simulink model "BaseEngineController_LS"  (Simulink 7.7)
settings: Solver=FixedStepDiscrete  StartTime=0.0  StopTime=10.0  RelTol=1e-3
PreLoadFcn:
  | try, eval([bdroot '_setup']); catch, eval('model_setup', ''); end
InitFcn:
  | try, eval([bdroot '_setup']); catch, eval('model_setup', ''); end
undefined symbols (not defined in the file): ECU555, High, motohawk_build_version, motohawk_trunc_name, motohawk_vardec_config_group, motohawk_vardec_path, True
libraries: MotoHawk_lib x1418, motohawk_control_primitives_lib x183, motohawk_engine_lib x32, simulink x21, motohawk_annotations_lib x9, AutoDoc_lib x8, simulink_extras x4, motohawk_ccp_examples_lib x1, motohawk_control_primitives_motoshare_lib x1
(part 17 of 27)

== system BaseEngineController_LS/Foreground/Control/VirtualSensors/RawProcessed/Capture ECT At Startup ==
  Signal_In : Inport
  Enable : EnablePort  StatesWhenEnabling=reset
  Add : Sum
  Add1 : Sum  Inputs=+-
  Collect Average : Subsystem  TreatAsAtomicUnit=on
  Constant : Constant  Value=int8(1)  SampleTime=-1
  Logical Operator : Logic  AllPortsSameDT=off  OutDataTypeStr=boolean
  Relational Operator : RelationalOperator  Operator=<=
  Relational Operator1 : RelationalOperator  Operator=>
  Sum : Sum  Inputs=++|  InputSameDT=on
  Switch : Switch  Threshold=1  ZeroCross=off  InputSameDT=on
  TwoSampleBuffer ToIgnore : Constant  Value=2  OutDataTypeStr=Inherit: Inherit via back propagation  SampleTime=-1
  Unit Delay : UnitDelay  SampleTime=-1
  motohawk_calibration : MotoHawk_lib/Calibration & Probing Blocks/motohawk_calibration  nam=[nam '_Count']  val=int8(count)  storage=Calibration  show_more=on  name_source=Use Parameter  data_type=Inherit from 'Default Value'  read_level=1  write_level=1  ovr_cals=on  view_as=Number  enum_struct={'Disabled', 'Enabled'}  vector_style=Wide Row  use_help_units=on  help='Number of samples to average at key-up to produce signal value'  units=''  use_header_enum=off  row_header_enum={}  col_header_enum={}  use_min_max=off  min_val=-inf  max_val=inf  use_precision=off  precision=''  gain=1  offset=0  exp=1  use_mototune_group=on  mototune_group=motohawk_vardec_path(gcb)
  motohawk_probe : MotoHawk_lib/Calibration & Probing Blocks/motohawk_probe  nam=nam  show_more=on  name_source=Use Parameter  read_level=1  view_as=Number  enum_struct={'Disabled', 'Enabled'}  vector_style=Wide Row  use_help_units=on  help=''  units=units  use_header_enum=off  row_header_enum={}  col_header_enum={}  use_precision=off  precision=''  gain=1  offset=0  exp=1  use_mototune_group=on  mototune_group=grp
  Signal_KeyUp : Outport
  wires:
  Sum/1 -> Switch/1, Relational Operator/1, Relational Operator1/1
  Relational Operator/1 -> Switch/2, Logical Operator/1
  Switch/1 -> Unit Delay/1, Add1/1
  Collect Average/1(Captured_Signal) -> motohawk_probe/1, Signal_KeyUp/1
  Signal_In/1 -> Collect Average/2(Signal)
  Unit Delay/1 -> Sum/1
  Constant/1 -> Sum/2
  motohawk_calibration/1 -> Add/1
  Add/1 -> Relational Operator/2, Switch/3
  TwoSampleBuffer ToIgnore/1 -> Add/2, Relational Operator1/2, Add1/2
  Logical Operator/1 -> Collect Average/Enable
  Relational Operator1/1 -> Logical Operator/2
  Add1/1 -> Collect Average/1(Count)

== system BaseEngineController_LS/Foreground/Control/VirtualSensors/RawProcessed/Capture IAT At Startup ==
  Signal_In : Inport
  Enable : EnablePort  StatesWhenEnabling=reset
  Add : Sum
  Add1 : Sum  Inputs=+-
  Collect Average : Subsystem  TreatAsAtomicUnit=on
  Constant : Constant  Value=int8(1)  SampleTime=-1
  Logical Operator : Logic  AllPortsSameDT=off  OutDataTypeStr=boolean
  Relational Operator : RelationalOperator  Operator=<=
  Relational Operator1 : RelationalOperator  Operator=>
  Sum : Sum  Inputs=++|  InputSameDT=on
  Switch : Switch  Threshold=1  ZeroCross=off  InputSameDT=on
  TwoSampleBuffer ToIgnore : Constant  Value=2  OutDataTypeStr=Inherit: Inherit via back propagation  SampleTime=-1
  Unit Delay : UnitDelay  SampleTime=-1
  motohawk_calibration : MotoHawk_lib/Calibration & Probing Blocks/motohawk_calibration  nam=[nam '_Count']  val=int8(count)  storage=Calibration  show_more=on  name_source=Use Parameter  data_type=Inherit from 'Default Value'  read_level=1  write_level=1  ovr_cals=on  view_as=Number  enum_struct={'Disabled', 'Enabled'}  vector_style=Wide Row  use_help_units=on  help='Number of samples to average at key-up to produce signal value'  units=''  use_header_enum=off  row_header_enum={}  col_header_enum={}  use_min_max=off  min_val=-inf  max_val=inf  use_precision=off  precision=''  gain=1  offset=0  exp=1  use_mototune_group=on  mototune_group=motohawk_vardec_path(gcb)
  motohawk_probe : MotoHawk_lib/Calibration & Probing Blocks/motohawk_probe  nam=nam  show_more=on  name_source=Use Parameter  read_level=1  view_as=Number  enum_struct={'Disabled', 'Enabled'}  vector_style=Wide Row  use_help_units=on  help=''  units=units  use_header_enum=off  row_header_enum={}  col_header_enum={}  use_precision=off  precision=''  gain=1  offset=0  exp=1  use_mototune_group=on  mototune_group=motohawk_vardec_path(gcb)
  Signal_KeyUp : Outport
  wires:
  Add1/1 -> Collect Average/1(Count)
  Relational Operator1/1 -> Logical Operator/2
  Logical Operator/1 -> Collect Average/Enable
  TwoSampleBuffer ToIgnore/1 -> Add1/2, Relational Operator1/2, Add/2
  Add/1 -> Switch/3, Relational Operator/2
  motohawk_calibration/1 -> Add/1
  Constant/1 -> Sum/2
  Unit Delay/1 -> Sum/1
  Signal_In/1 -> Collect Average/2(Signal)
  Collect Average/1(Captured_Signal) -> Signal_KeyUp/1, motohawk_probe/1
  Switch/1 -> Add1/1, Unit Delay/1
  Relational Operator/1 -> Logical Operator/1, Switch/2
  Sum/1 -> Relational Operator1/1, Relational Operator/1, Switch/1

== system BaseEngineController_LS/Foreground/Control/VirtualSensors/RawProcessed/CutThrottle APP Limiting ==
  APP_in [%] : Inport
  Bound APP if overheating : motohawk_control_primitives_lib/Saturation  SystemSampleTime=-1
  Constant1 : Constant  Value=0  SampleTime=-1
  Data Type Conversion : DataTypeConversion  OutDataTypeStr=double
  Product1 : Product  RndMeth=Zero
  Switch1 : Switch  Threshold=1
  motohawk_calibration1 : MotoHawk_lib/Calibration & Probing Blocks/motohawk_calibration  nam='Overheat_MaxAPP'  val=10  storage=Calibration  show_more=on  name_source=Use Parameter  data_type=uint8  read_level=1  write_level=1  ovr_cals=on  view_as=Number  enum_struct={'Disabled', 'Enabled'}  vector_style=Wide Row  use_help_units=on  help='Max APP command to allow during overheat condition'  units='%'  use_header_enum=off  row_header_enum={}  col_header_enum={}  use_min_max=on  min_val=-inf  max_val=inf  use_precision=off  precision=''  gain=1  offset=0  exp=1  use_mototune_group=on  mototune_group=motohawk_vardec_path(gcb)
  motohawk_calibration2 : MotoHawk_lib/Calibration & Probing Blocks/motohawk_calibration  nam='Overheat_ScaleAPP'  val=0.1  storage=Calibration  show_more=on  name_source=Use Parameter  data_type=double  read_level=1  write_level=1  ovr_cals=on  view_as=Number  enum_struct={'Disabled', 'Enabled'}  vector_style=Wide Row  use_help_units=on  help='Scale APP by this factor when overheating'  units='multiplier'  use_header_enum=off  row_header_enum={}  col_header_enum={}  use_min_max=on  min_val=-inf  max_val=inf  use_precision=off  precision=''  gain=1  offset=0  exp=1  use_mototune_group=on  mototune_group=motohawk_vardec_path(gcb)
  motohawk_fault_action1 : MotoHawk_lib/Fault Management Blocks/motohawk_fault_action  nam='CutThrottle'  output_status=on  eval_nam=CutThrottle
  APP_out [%] : Outport
  wires:
  APP_in [%]/1 -> Switch1/3, Product1/2
  Product1/1 -> Bound APP if overheating/1
  motohawk_fault_action1/1 -> Switch1/2
  Constant1/1 -> Bound APP if overheating/2
  Bound APP if overheating/1 -> Switch1/1
  motohawk_calibration2/1 -> Product1/1
  Switch1/1 -> APP_out [%]/1
  motohawk_calibration1/1 -> Data Type Conversion/1
  Data Type Conversion/1 -> Bound APP if overheating/3

== system BaseEngineController_LS/Foreground/Control/VirtualSensors/RawProcessed/Engine Accel ==
  RPM : Inport
  Derivitive3 : motohawk_control_primitives_lib/Derivitive  SystemSampleTime=-1  samp_time=-1
  First Order Low Pass (Tunable) : motohawk_control_primitives_lib/First Order Low Pass (Tunable)  SystemSampleTime=-1  nam='EngineAccelFiltConst'  samp_time=.005  group=motohawk_vardec_path(gcb)
  motohawk_probe1 : MotoHawk_lib/Calibration & Probing Blocks/motohawk_probe  nam='EngineAccel'  show_more=on  name_source=Use Parameter  read_level=1  view_as=Number  enum_struct={'Disabled', 'Enabled'}  vector_style=Wide Row  use_help_units=on  help='Acceleration rate of engine'  units='RPM/s'  use_header_enum=off  row_header_enum={}  col_header_enum={}  use_precision=on  precision=''  gain=1  offset=0  exp=1  use_mototune_group=on  mototune_group=motohawk_vardec_path(gcb)
  RPM Accel : Outport
  wires:
  First Order Low Pass (Tunable)/1 -> RPM Accel/1, motohawk_probe1/1
  RPM/1 -> Derivitive3/1
  Derivitive3/1 -> First Order Low Pass (Tunable)/1

== system BaseEngineController_LS/Foreground/Control/VirtualSensors/RawProcessed/EngineState ==
  note: States:
      | 1 - Stall
      | 2 - Crank
      | 3 - Run
  RPM : Inport
  Data Type Conversion : DataTypeConversion  SaturateOnIntegerOverflow=on  RndMeth=Zero
  Engine State Machine : Stateflow chart  TreatAsAtomicUnit=on
  Logical Operator1 : Logic
  Relational Operator1 : RelationalOperator  Operator=<  ZeroCross=off  InputSameDT=on
  Relational Operator2 : RelationalOperator  Operator=>  ZeroCross=off  InputSameDT=on
  Relational Operator3 : RelationalOperator  ZeroCross=off  InputSameDT=on
  Relational Operator4 : RelationalOperator  Operator=>  ZeroCross=off  InputSameDT=on
  Sum : Sum  Inputs=|-+  SaturateOnIntegerOverflow=on
  TDC_Counter : Subsystem  TreatAsAtomicUnit=on
  Unit Delay : UnitDelay  SampleTime=-1
  motohawk_calibration1 : MotoHawk_lib/Calibration & Probing Blocks/motohawk_calibration  nam='CrankToRunRPMThresh'  val=500  storage=Calibration  show_more=on  name_source=Use Parameter  data_type=uint16  read_level=1  write_level=1  ovr_cals=on  view_as=Number  enum_struct={'Disabled', 'Enabled'}  vector_style=Wide Row  use_help_units=on  help='RPM above which RUN mode can be entered from CRANK mode.'  units='RPM'  use_header_enum=off  row_header_enum={}  col_header_enum={}  use_min_max=off  min_val=0  max_val=inf  use_precision=off  precision=''  gain=1  offset=0  exp=1  use_mototune_group=on  mototune_group=motohawk_vardec_path(gcb)
  motohawk_calibration2 : MotoHawk_lib/Calibration & Probing Blocks/motohawk_calibration  nam='RunLatchTDCs'  val=4  storage=Calibration  show_more=on  name_source=Use Parameter  data_type=uint8  read_level=1  write_level=1  ovr_cals=on  view_as=Number  enum_struct={'Disabled', 'Enabled'}  vector_style=Wide Row  use_help_units=on  help='Number of TDCs required to be above CrankToRunRPMThresh before the RUN mode is invoked.'  units='TDCs'  use_header_enum=off  row_header_enum={}  col_header_enum={}  use_min_max=off  min_val=0  max_val=inf  use_precision=off  precision=''  gain=1  offset=0  exp=1  use_mototune_group=on  mototune_group=motohawk_vardec_path(gcb)
  motohawk_calibration3 : MotoHawk_lib/Calibration & Probing Blocks/motohawk_calibration  nam='StallRPMThresholdHyst'  val=10  storage=Calibration  show_more=on  name_source=Use Parameter  data_type=uint16  read_level=1  write_level=1  ovr_cals=on  view_as=Number  enum_struct={'Disabled', 'Enabled'}  vector_style=Wide Row  use_help_units=on  help='Hysteresis used in conjunction with Min. RPM Threshold to determine when engine state transition to STALL. '  units='RPM'  use_header_enum=off  row_header_enum={}  col_header_enum={}  use_min_max=off  min_val=0  max_val=inf  use_precision=off  precision=''  gain=1  offset=0  exp=1  use_mototune_group=on  mototune_group=motohawk_vardec_path(gcb)
  motohawk_calibration4 : MotoHawk_lib/Calibration & Probing Blocks/motohawk_calibration  nam='StallRPMMinThreshold'  val=50  storage=Calibration  show_more=on  name_source=Use Parameter  data_type=uint16  read_level=1  write_level=1  ovr_cals=on  view_as=Number  enum_struct={'Disabled', 'Enabled'}  vector_style=Wide Row  use_help_units=on  help='Min. RPM Threshold below which engine state transition to STALL.'  units='RPM'  use_header_enum=off  row_header_enum={}  col_header_enum={}  use_min_max=on  min_val=0  max_val=inf  use_precision=off  precision=''  gain=1  offset=0  exp=1  use_mototune_group=on  mototune_group=motohawk_vardec_path(gcb)
  motohawk_data_def : MotoHawk_lib/Data Storage Blocks/motohawk_data_def  nam='EngineState'  container_nam=''  data=0  typ=uint8  struct_nam='MyStruct'  storage=Volatile  outputRef=off  use_vardec=off  window=Display  read_level=1  write_level=1  ovr_cals=on  view_as=Enumeration  enum_struct={'', 'Stall', 'Crank', 'Run'}  vector_style=Wide Row  use_help_units=on  help='Engine state based on RPM.'  units=''  use_header_enum=off  row_header_enum={}  col_header_enum={}  use_min_max=on  min_val=-inf  max_val=inf  use_precision=off  precision=''  gain=1  offset=0  exp=1  use_mototune_group=on  mototune_group=motohawk_vardec_path(gcb)  eval_name=EngineState  data_stores=motohawk_sfun_data_def_data_stores  struct_instances=motohawk_sfun_data_def_struct_instances  vardecs=motohawk_sfun_data_def_vardecs
  motohawk_data_write : MotoHawk_lib/Data Storage Blocks/motohawk_data_write  source=Lookup By Name  structure=Scalar  operation=Write entire data structure at once  sz_vec=-1  sz_row=3  sz_col=2  typ=uint8  nam='EngineState'  checkNull=off  write_read_only=off  struct_inst_name='Struct1'  struct_name='MyStruct'
  motohawk_probe : MotoHawk_lib/Calibration & Probing Blocks/motohawk_probe  nam='EngineStateRaw'  show_more=on  name_source=Use Parameter  read_level=1  view_as=Number  enum_struct={'Disabled', 'Enabled'}  vector_style=Wide Row  use_help_units=off  help=''  units=''  use_header_enum=off  row_header_enum={}  col_header_enum={}  use_precision=off  precision=''  gain=1  offset=0  exp=1  use_mototune_group=on  mototune_group=motohawk_vardec_path(gcb)
  motohawk_probe2 : MotoHawk_lib/Calibration & Probing Blocks/motohawk_probe  nam='CrankTrans'  show_more=on  name_source=Use Parameter  read_level=1  view_as=Number  enum_struct={'Disabled', 'Enabled'}  vector_style=Wide Row  use_help_units=off  help=''  units=''  use_header_enum=off  row_header_enum={}  col_header_enum={}  use_precision=off  precision=''  gain=1  offset=0  exp=1  use_mototune_group=on  mototune_group=motohawk_vardec_path(gcb)
  motohawk_trigger : MotoHawk_lib/Trigger Blocks/motohawk_trigger  Tag=Trigger  trigger=FGND_TDC_EVENT  function_name=Trigger_FGND_TDC_EVENT_3098p0051  priority_order=0  inherited=on  run_disabled=off  override_app_monitor=off  target=ECU555_80
  State : Outport
  wires:
  motohawk_calibration4/1 -> Relational Operator4/2, Sum/2
  Relational Operator4/1 -> Engine State Machine/2(Crank), motohawk_probe2/1  "Crank"
  Data Type Conversion/1 -> Relational Operator1/1, Relational Operator4/1, Relational Operator2/1
  RPM/1 -> Data Type Conversion/1  "RPM"
  Relational Operator1/1 -> Engine State Machine/1(Stall)  "Stall"
  Engine State Machine/1(State) -> State/1, Unit Delay/1, motohawk_probe/1, motohawk_data_write/1
  Relational Operator2/1 -> Logical Operator1/1
  Relational Operator3/1 -> Logical Operator1/2
  Logical Operator1/1 -> Engine State Machine/3(Run)  "Run"
  motohawk_trigger/1 -> TDC_Counter/Trigger
  TDC_Counter/1(CrankCount) -> Relational Operator3/1
  Unit Delay/1 -> TDC_Counter/1(State)
  motohawk_calibration3/1 -> Sum/1
  Sum/1 -> Relational Operator1/2
  motohawk_calibration1/1 -> Relational Operator2/2
  motohawk_calibration2/1 -> Relational Operator3/2

== system BaseEngineController_LS/Foreground/Control/VirtualSensors/RawProcessed/Fuel Delta Pressure Calculation ==
  FuelPressure : Inport
  "MAP " : Inport  Port=2
  Sum3 : Sum  Inputs=++-  SaturateOnIntegerOverflow=on
  kPa Gauge to kPa absolute : Constant  Value=100  SampleTime=-1
  motohawk_probe : MotoHawk_lib/Calibration & Probing Blocks/motohawk_probe  nam='FuelDeltaPressure'  show_more=on  name_source=Use Parameter  read_level=1  view_as=Number  enum_struct={'Disabled', 'Enabled'}  vector_style=Wide Row  use_help_units=on  help='Fuel pressure across injector (rail - manifold)'  units='kPa'  use_header_enum=off  row_header_enum={}  col_header_enum={}  use_precision=on  precision=''  gain=1  offset=0  exp=1  use_mototune_group=on  mototune_group=motohawk_vardec_path(gcb)
  "FuelDeltaPressure " : Outport
  wires:
  FuelPressure/1 -> Sum3/1
  "MAP "/1 -> Sum3/3
  Sum3/1 -> "FuelDeltaPressure "/1, motohawk_probe/1
  kPa Gauge to kPa absolute/1 -> Sum3/2

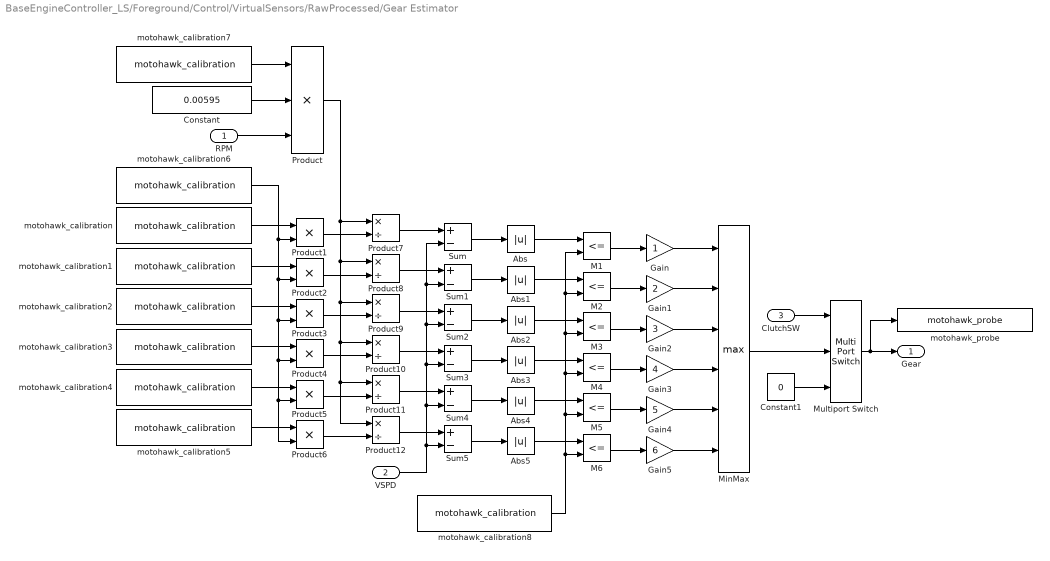
== system BaseEngineController_LS/Foreground/Control/VirtualSensors/RawProcessed/Gear Estimator ==
  RPM : Inport
  VSPD : Inport  Port=2
  ClutchSW : Inport  Port=3
  Abs{,1..5} (6 alike) : Abs
  Constant : Constant  Value=0.00595
  Constant1 : Constant  Value=0
  Gain : Gain
  Gain1 : Gain  Gain=2
  Gain2 : Gain  Gain=3
  Gain3 : Gain  Gain=4
  Gain4 : Gain  Gain=5
  Gain5 : Gain  Gain=6
  M{1..6} (6 alike) : RelationalOperator  Operator=<=  OutDataTypeStr=boolean
  MinMax : MinMax  Function=max  Inputs=6
  Multiport Switch : MultiPortSwitch  DataPortOrder=Zero-based contiguous  Inputs=2  zeroidx=on
  Product : Product  Inputs=***  RndMeth=Zero
  Product{1..6} (6 alike) : Product  RndMeth=Zero
  Product{7..12} (6 alike) : Product  Inputs=*/  RndMeth=Zero
  Sum{,1..5} (6 alike) : Sum  Inputs=+-
  motohawk_calibration : MotoHawk_lib/Calibration & Probing Blocks/motohawk_calibration  nam='Gear1Ratio'  val=2.97  storage=Calibration  show_more=on  name_source=Use Parameter  data_type=Inherit from 'Default Value'  read_level=1  write_level=1  ovr_cals=on  view_as=Number  enum_struct={'Disabled', 'Enabled'}  vector_style=Wide Row  use_help_units=off  help=''  units=''  use_header_enum=off  row_header_enum={}  col_header_enum={}  use_min_max=off  min_val=-inf  max_val=inf  use_precision=off  precision=''  gain=1  offset=0  exp=1  use_mototune_group=off  mototune_group=motohawk_vardec_path(gcb)
  motohawk_calibration1 : MotoHawk_lib/Calibration & Probing Blocks/motohawk_calibration  nam='Gear2Ratio'  val=2.07  storage=Calibration  show_more=on  name_source=Use Parameter  data_type=Inherit from 'Default Value'  read_level=1  write_level=1  ovr_cals=on  view_as=Number  enum_struct={'Disabled', 'Enabled'}  vector_style=Wide Row  use_help_units=off  help=''  units=''  use_header_enum=off  row_header_enum={}  col_header_enum={}  use_min_max=off  min_val=-inf  max_val=inf  use_precision=off  precision=''  gain=1  offset=0  exp=1  use_mototune_group=off  mototune_group=motohawk_vardec_path(gcb)
  motohawk_calibration2 : MotoHawk_lib/Calibration & Probing Blocks/motohawk_calibration  nam='Gear3Ratio'  val=1.43  storage=Calibration  show_more=on  name_source=Use Parameter  data_type=Inherit from 'Default Value'  read_level=1  write_level=1  ovr_cals=on  view_as=Number  enum_struct={'Disabled', 'Enabled'}  vector_style=Wide Row  use_help_units=off  help=''  units=''  use_header_enum=off  row_header_enum={}  col_header_enum={}  use_min_max=off  min_val=-inf  max_val=inf  use_precision=off  precision=''  gain=1  offset=0  exp=1  use_mototune_group=off  mototune_group=motohawk_vardec_path(gcb)
  motohawk_calibration3 : MotoHawk_lib/Calibration & Probing Blocks/motohawk_calibration  nam='Gear4Ratio'  val=1  storage=Calibration  show_more=on  name_source=Use Parameter  data_type=Inherit from 'Default Value'  read_level=1  write_level=1  ovr_cals=on  view_as=Number  enum_struct={'Disabled', 'Enabled'}  vector_style=Wide Row  use_help_units=off  help=''  units=''  use_header_enum=off  row_header_enum={}  col_header_enum={}  use_min_max=off  min_val=-inf  max_val=inf  use_precision=off  precision=''  gain=1  offset=0  exp=1  use_mototune_group=off  mototune_group=motohawk_vardec_path(gcb)
  motohawk_calibration4 : MotoHawk_lib/Calibration & Probing Blocks/motohawk_calibration  nam='Gear5Ratio'  val=0.84  storage=Calibration  show_more=on  name_source=Use Parameter  data_type=Inherit from 'Default Value'  read_level=1  write_level=1  ovr_cals=on  view_as=Number  enum_struct={'Disabled', 'Enabled'}  vector_style=Wide Row  use_help_units=off  help=''  units=''  use_header_enum=off  row_header_enum={}  col_header_enum={}  use_min_max=off  min_val=-inf  max_val=inf  use_precision=off  precision=''  gain=1  offset=0  exp=1  use_mototune_group=off  mototune_group=motohawk_vardec_path(gcb)
  motohawk_calibration5 : MotoHawk_lib/Calibration & Probing Blocks/motohawk_calibration  nam='Gear6Ratio'  val=0.56  storage=Calibration  show_more=on  name_source=Use Parameter  data_type=Inherit from 'Default Value'  read_level=1  write_level=1  ovr_cals=on  view_as=Number  enum_struct={'Disabled', 'Enabled'}  vector_style=Wide Row  use_help_units=off  help=''  units=''  use_header_enum=off  row_header_enum={}  col_header_enum={}  use_min_max=off  min_val=-inf  max_val=inf  use_precision=off  precision=''  gain=1  offset=0  exp=1  use_mototune_group=off  mototune_group=motohawk_vardec_path(gcb)
  motohawk_calibration6 : MotoHawk_lib/Calibration & Probing Blocks/motohawk_calibration  nam='FDR'  val=4.73  storage=Calibration  show_more=on  name_source=Use Parameter  data_type=Inherit from 'Default Value'  read_level=1  write_level=1  ovr_cals=on  view_as=Number  enum_struct={'Disabled', 'Enabled'}  vector_style=Wide Row  use_help_units=off  help=''  units=''  use_header_enum=off  row_header_enum={}  col_header_enum={}  use_min_max=off  min_val=-inf  max_val=inf  use_precision=off  precision=''  gain=1  offset=0  exp=1  use_mototune_group=off  mototune_group=motohawk_vardec_path(gcb)
  motohawk_calibration7 : MotoHawk_lib/Calibration & Probing Blocks/motohawk_calibration  nam='TireRadius'  val=10  storage=Calibration  show_more=on  name_source=Use Parameter  data_type=Inherit from 'Default Value'  read_level=1  write_level=1  ovr_cals=on  view_as=Number  enum_struct={'Disabled', 'Enabled'}  vector_style=Wide Row  use_help_units=off  help=''  units=''  use_header_enum=off  row_header_enum={}  col_header_enum={}  use_min_max=off  min_val=-inf  max_val=inf  use_precision=off  precision=''  gain=1  offset=0  exp=1  use_mototune_group=off  mototune_group=motohawk_vardec_path(gcb)
  motohawk_calibration8 : MotoHawk_lib/Calibration & Probing Blocks/motohawk_calibration  nam='GearMatchHyst'  val=2  storage=Calibration  show_more=off  name_source=Use Parameter  data_type=Inherit from 'Default Value'  read_level=1  write_level=1  ovr_cals=on  view_as=Number  enum_struct={'Disabled', 'Enabled'}  vector_style=Wide Row  use_help_units=off  help=''  units=''  use_header_enum=off  row_header_enum={}  col_header_enum={}  use_min_max=off  min_val=-inf  max_val=inf  use_precision=off  precision=''  gain=1  offset=0  exp=1  use_mototune_group=off  mototune_group=motohawk_vardec_path(gcb)
  motohawk_probe : MotoHawk_lib/Calibration & Probing Blocks/motohawk_probe  nam='GearEstimated'  show_more=off  name_source=Use Parameter  read_level=1  view_as=Number  enum_struct={'Disabled', 'Enabled'}  vector_style=Wide Row  use_help_units=off  help=''  units=''  use_header_enum=off  row_header_enum={}  col_header_enum={}  use_precision=off  precision=''  gain=1  offset=0  exp=1  use_mototune_group=off  mototune_group=motohawk_vardec_path(gcb)
  Gear : Outport
  wires:
  motohawk_calibration7/1 -> Product/1
  RPM/1 -> Product/3
  Constant/1 -> Product/2
  motohawk_calibration/1 -> Product1/1
  motohawk_calibration6/1 -> Product1/2, Product2/2, Product3/2, Product4/2, Product6/2, Product5/2
  motohawk_calibration1/1 -> Product2/1
  motohawk_calibration2/1 -> Product3/1
  motohawk_calibration3/1 -> Product4/1
  motohawk_calibration4/1 -> Product5/1
  motohawk_calibration5/1 -> Product6/1
  Product1/1 -> Product7/2
  Product/1 -> Product7/1, Product8/1, Product9/1, Product10/1, Product11/1, Product12/1
  Product2/1 -> Product8/2
  Product3/1 -> Product9/2
  Product4/1 -> Product10/2
  Product5/1 -> Product11/2
  Product6/1 -> Product12/2
  Product7/1 -> Sum/1
  Product8/1 -> Sum1/1
  Product9/1 -> Sum2/1
  Product10/1 -> Sum3/1
  Product11/1 -> Sum4/1
  Product12/1 -> Sum5/1
  VSPD/1 -> Sum/2, Sum1/2, Sum2/2, Sum3/2, Sum4/2, Sum5/2
  Sum/1 -> Abs/1
  Sum1/1 -> Abs1/1
  Sum2/1 -> Abs2/1
  Sum3/1 -> Abs3/1
  Sum4/1 -> Abs4/1
  Sum5/1 -> Abs5/1
  Abs/1 -> M1/1
  Abs1/1 -> M2/1
  Abs2/1 -> M3/1
  Abs3/1 -> M4/1
  Abs4/1 -> M5/1
  Abs5/1 -> M6/1
  motohawk_calibration8/1 -> M1/2, M2/2, M3/2, M4/2, M5/2, M6/2
  M1/1 -> Gain/1
  M2/1 -> Gain1/1
  M3/1 -> Gain2/1
  M4/1 -> Gain3/1
  M5/1 -> Gain4/1
  M6/1 -> Gain5/1
  Gain/1 -> MinMax/1
  Gain1/1 -> MinMax/2
  Gain2/1 -> MinMax/3
  Gain3/1 -> MinMax/4
  Gain4/1 -> MinMax/5
  Gain5/1 -> MinMax/6
  MinMax/1 -> Multiport Switch/2
  ClutchSW/1 -> Multiport Switch/1
  Constant1/1 -> Multiport Switch/3
  Multiport Switch/1 -> Gear/1, motohawk_probe/1

== system BaseEngineController_LS/Foreground/Control/VirtualSensors/RawProcessed/O2 De-lag ==
  O2_BankA : Inport
  O2_BankB : Inport  Port=2
  Constant : Constant
  Constant1 : Constant
  Product{,1..3} (4 alike) : Product  RndMeth=Zero
  Sum : Sum  Inputs=|+-
  Sum1 : Sum  Inputs=+|+
  Sum2 : Sum  Inputs=|+-
  Sum3 : Sum  Inputs=+|+
  Unit Delay : UnitDelay  SampleTime=-1
  Unit Delay1 : UnitDelay  SampleTime=-1
  motohawk_calibration : MotoHawk_lib/Calibration & Probing Blocks/motohawk_calibration  nam='O2BankA_DelagFilterConst'  val=0.05  storage=Calibration  show_more=on  name_source=Use Parameter  data_type=Inherit from 'Default Value'  read_level=1  write_level=1  ovr_cals=on  view_as=Number  enum_struct={'Disabled', 'Enabled'}  vector_style=Wide Row  use_help_units=on  help='First-order filter time constant of the pre-catalyst O2 signal.'  units='s'  use_header_enum=off  row_header_enum={}  col_header_enum={}  use_min_max=off  min_val=-inf  max_val=inf  use_precision=off  precision=''  gain=1  offset=0  exp=1  use_mototune_group=on  mototune_group=motohawk_vardec_path(gcb)
  motohawk_calibration1 : MotoHawk_lib/Calibration & Probing Blocks/motohawk_calibration  nam='O2BankB_DelagFiltConst'  val=0.05  storage=Calibration  show_more=on  name_source=Use Parameter  data_type=Inherit from 'Default Value'  read_level=1  write_level=1  ovr_cals=on  view_as=Number  enum_struct={'Disabled', 'Enabled'}  vector_style=Wide Row  use_help_units=on  help='First-order filter time constant of the post-catalyst O2 signal.'  units='s'  use_header_enum=off  row_header_enum={}  col_header_enum={}  use_min_max=off  min_val=-inf  max_val=inf  use_precision=off  precision=''  gain=1  offset=0  exp=1  use_mototune_group=on  mototune_group=motohawk_vardec_path(gcb)
  motohawk_probe : MotoHawk_lib/Calibration & Probing Blocks/motohawk_probe  nam='O2BankA_O2Delag'  show_more=on  name_source=Use Parameter  read_level=1  view_as=Number  enum_struct={'Disabled', 'Enabled'}  vector_style=Wide Row  use_help_units=on  help=''  units=''  use_header_enum=off  row_header_enum={}  col_header_enum={}  use_precision=on  precision=''  gain=1  offset=0  exp=1  use_mototune_group=on  mototune_group=motohawk_vardec_path(gcb)
  motohawk_probe1 : MotoHawk_lib/Calibration & Probing Blocks/motohawk_probe  nam='O2BankB_O2Delag'  show_more=on  name_source=Use Parameter  read_level=1  view_as=Number  enum_struct={'Disabled', 'Enabled'}  vector_style=Wide Row  use_help_units=on  help=''  units=''  use_header_enum=off  row_header_enum={}  col_header_enum={}  use_precision=on  precision=''  gain=1  offset=0  exp=1  use_mototune_group=on  mototune_group=motohawk_vardec_path(gcb)
  O2BankADelagged : Outport
  O2BankBDelagged : Outport  Port=2
  wires:
  motohawk_calibration/1 -> Product/1, Sum/2
  O2_BankA/1 -> Product/2, Unit Delay/1
  Constant/1 -> Sum/1
  Unit Delay/1 -> Product1/1
  Sum/1 -> Product1/2
  Product/1 -> Sum1/2
  Product1/1 -> Sum1/1
  Sum1/1 -> O2BankADelagged/1, motohawk_probe/1
  motohawk_calibration1/1 -> Sum2/2, Product2/1
  O2_BankB/1 -> Unit Delay1/1, Product2/2
  Constant1/1 -> Sum2/1
  Unit Delay1/1 -> Product3/1
  Sum2/1 -> Product3/2
  Product2/1 -> Sum3/2
  Product3/1 -> Sum3/1
  Sum3/1 -> motohawk_probe1/1, O2BankBDelagged/1

== system BaseEngineController_LS/Foreground/Control/VirtualSensors/RawProcessed/TPS  Sensor Arbitration ==
  note: Normally take TPS1
      | If TPS1 faulted, take TPS2
      | If both are faulted, take the larger
      | of the two to force ETC controller
      | to zero.
  note: Normally APP1
  TPS1 : Inport
  TPS2 : Inport  Port=2
  Abs : Abs  SaturateOnIntegerOverflow=on
  Logical Operator1 : Logic  Operator=OR  AllPortsSameDT=off
  Logical Operator4 : Logic  Operator=OR  AllPortsSameDT=off
  Logical Operator5 : Logic  Operator=OR  AllPortsSameDT=off
  Logical Operator6 : Logic  AllPortsSameDT=off
  MinMax : MinMax  Function=max  Inputs=2
  Relational Operator3 : RelationalOperator  Operator=>  OutDataTypeStr=boolean
  Sum : Sum  Inputs=|+-  SaturateOnIntegerOverflow=on
  Switch1 : Switch  Threshold=1  SaturateOnIntegerOverflow=on
  Switch2 : Switch  Threshold=1  SaturateOnIntegerOverflow=on
  motohawk_calibration2 : MotoHawk_lib/Calibration & Probing Blocks/motohawk_calibration  nam='TPS1_TPS2_Max_Deviation'  val=100  storage=Calibration  show_more=on  name_source=Use Parameter  data_type=double  read_level=1  write_level=1  ovr_cals=on  view_as=Number  enum_struct={'Disabled', 'Enabled'}  vector_style=Wide Row  use_help_units=on  help='Specifies the maximum allowable deviation between the two sensors'  units='Percent'  use_header_enum=off  row_header_enum={}  col_header_enum={}  use_min_max=off  min_val=-inf  max_val=inf  use_precision=off  precision=''  gain=1  offset=0  exp=1  use_mototune_group=on  mototune_group=motohawk_vardec_path(gcb)
  motohawk_fault_def1 : MotoHawk_lib/Fault Management Blocks/motohawk_fault_def  nam='TPS_Sensors_Conflict'  mode=Enabled  id=[]  x=25  y=50  input_suspected=on  indeterminate=off  increment_xy=on  downsample_count=1  ovr_cals=on  ovr_actions=on  show_actions=off  action1_name=''  action1_cond=(None)  action2_name=''  action2_cond=(None)  action3_name=''  action3_cond=(None)  action4_name=''  action4_cond=(None)
  motohawk_fault_status : MotoHawk_lib/Fault Management Blocks/motohawk_fault_status  source=Lookup By Name  nam='TPS1RangeHigh'  status=Active
  motohawk_fault_status1 : MotoHawk_lib/Fault Management Blocks/motohawk_fault_status  source=Lookup By Name  nam='TPS1RangeLow'  status=Active
  motohawk_fault_status2 : MotoHawk_lib/Fault Management Blocks/motohawk_fault_status  source=Lookup By Name  nam='TPS2RangeLow'  status=Active
  motohawk_fault_status3 : MotoHawk_lib/Fault Management Blocks/motohawk_fault_status  source=Lookup By Name  nam='TPS2RangeHigh'  status=Active
  motohawk_fault_status4 : MotoHawk_lib/Fault Management Blocks/motohawk_fault_status  source=Lookup By Name  nam='TPS_Sensors_Conflict'  status=Active
  motohawk_probe : MotoHawk_lib/Calibration & Probing Blocks/motohawk_probe  nam='TPSFinal'  show_more=on  name_source=Use Parameter  read_level=1  view_as=Number  enum_struct={'Disabled', 'Enabled'}  vector_style=Wide Row  use_help_units=on  help=''  units='%'  use_header_enum=off  row_header_enum={}  col_header_enum={}  use_precision=off  precision=''  gain=1  offset=0  exp=1  use_mototune_group=off  mototune_group=motohawk_vardec_path(gcb)
  TPS : Outport
  wires:
  Sum/1 -> Abs/1
  Abs/1 -> Relational Operator3/1
  motohawk_calibration2/1 -> Relational Operator3/2
  TPS1/1 -> Sum/1, Switch1/3, MinMax/2
  TPS2/1 -> Sum/2, Switch1/1, MinMax/1
  Relational Operator3/1 -> motohawk_fault_def1/1
  motohawk_fault_status/1 -> Logical Operator4/1
  motohawk_fault_status1/1 -> Logical Operator4/2
  motohawk_fault_status3/1 -> Logical Operator5/1
  motohawk_fault_status2/1 -> Logical Operator5/2
  Switch2/1 -> TPS/1, motohawk_probe/1
  Logical Operator4/1 -> Switch1/2, Logical Operator6/1
  Logical Operator5/1 -> Logical Operator6/2
  Switch1/1 -> Switch2/3
  Logical Operator6/1 -> Logical Operator1/1  "Both Faulted"
  motohawk_fault_status4/1 -> Logical Operator1/2
  MinMax/1 -> Switch2/1
  Logical Operator1/1 -> Switch2/2

== system BaseEngineController_LS/Foreground/Control/VirtualSensors/RawProcessed/Time Since Key On ==
  Constant : Constant  Value=true
  Time Since Enabled (With Input)2 : motohawk_control_primitives_lib/Time Since Enabled (With Input)1  SystemSampleTime=-1  nam='TimeSinceKeyOnTimer'  samp_time=-1  init=0  upperlim=16000
  motohawk_probe : MotoHawk_lib/Calibration & Probing Blocks/motohawk_probe  nam='TimeSinceKeyOn'  show_more=on  name_source=Use Parameter  read_level=1  view_as=Number  enum_struct={'Disabled', 'Enabled'}  vector_style=Wide Row  use_help_units=off  help=''  units=''  use_header_enum=off  row_header_enum={}  col_header_enum={}  use_precision=off  precision=''  gain=1  offset=0  exp=1  use_mototune_group=on  mototune_group=motohawk_vardec_path(gcb)
  Time : Outport
  wires:
  Constant/1 -> Time Since Enabled (With Input)2/1
  Time Since Enabled (With Input)2/1 -> Time/1, motohawk_probe/1

== system BaseEngineController_LS/Foreground/Control/VirtualSensors/RawProcessed/Time Since Run ==
  RunState : motohawk_control_primitives_lib/CompareTo  SystemSampleTime=-1  op===  val=3
  Time Since Enabled (With Input)2 : motohawk_control_primitives_lib/Time Since Enabled (With Input)1  SystemSampleTime=-1  nam='TimeSinceRunTimer'  samp_time=-1  init=0  upperlim=16000
  motohawk_data_read : MotoHawk_lib/Data Storage Blocks/motohawk_data_read  source=Lookup By Name  structure=Scalar  operation=Read entire data structure at once  sz_vec=4  sz_row=2  sz_col=3  typ=uint8  nam='EngineState'  checkNull=on  struct_inst_name='Struct1'  struct_nam='MyStruct'
  motohawk_probe : MotoHawk_lib/Calibration & Probing Blocks/motohawk_probe  nam='TimeSinceRun'  show_more=on  name_source=Use Parameter  read_level=1  view_as=Number  enum_struct={'Disabled', 'Enabled'}  vector_style=Wide Row  use_help_units=off  help=''  units=''  use_header_enum=off  row_header_enum={}  col_header_enum={}  use_precision=off  precision=''  gain=1  offset=0  exp=1  use_mototune_group=on  mototune_group=motohawk_vardec_path(gcb)
  Time : Outport
  wires:
  RunState/1 -> Time Since Enabled (With Input)2/1
  Time Since Enabled (With Input)2/1 -> motohawk_probe/1, Time/1
  motohawk_data_read/1 -> RunState/1

== system BaseEngineController_LS/Foreground/Control/VirtualSensors/RawProcessed/Time Since Stall ==
  Constant1 : Constant  Value=150  OutDataTypeStr=Inherit: Inherit via back propagation  SampleTime=-1
  Logical Operator : Logic  AllPortsSameDT=off  OutDataTypeStr=boolean
  Relational Operator : RelationalOperator  Operator=>  ZeroCross=off  InputSameDT=on
  Stall State : motohawk_control_primitives_lib/CompareTo  SystemSampleTime=-1  op===  val=1
  Time Since Enabled (With Input)1 : motohawk_control_primitives_lib/Time Since Enabled (With Input)1  SystemSampleTime=-1  nam='TimeSinceStallTimer'  samp_time=-1  init=0  upperlim=16000
  motohawk_ain_read : MotoHawk_lib/Analog I//O Blocks/motohawk_ain_read  nam='ECUP'  typ=uint16
  motohawk_data_read : MotoHawk_lib/Data Storage Blocks/motohawk_data_read  source=Lookup By Name  structure=Scalar  operation=Read entire data structure at once  sz_vec=4  sz_row=2  sz_col=3  typ=uint8  nam='EngineState'  checkNull=on  struct_inst_name='Struct1'  struct_nam='MyStruct'
  motohawk_probe : MotoHawk_lib/Calibration & Probing Blocks/motohawk_probe  nam='TimeSinceStall'  show_more=on  name_source=Use Parameter  read_level=1  view_as=Number  enum_struct={'Open-Loop', 'Closed-Loop'}  vector_style=Wide Row  use_help_units=on  help='Indicates time since entering Stall State - saturates and disables at 2000 seconds'  units='s'  use_header_enum=off  row_header_enum={}  col_header_enum={}  use_precision=off  precision=''  gain=1  offset=0  exp=1  use_mototune_group=on  mototune_group=motohawk_vardec_path(gcb)
  Time : Outport
  wires:
  Logical Operator/1 -> Time Since Enabled (With Input)1/1
  Time Since Enabled (With Input)1/1 -> Time/1, motohawk_probe/1
  motohawk_data_read/1 -> Stall State/1
  motohawk_ain_read/1 -> Relational Operator/1
  Constant1/1 -> Relational Operator/2
  Stall State/1 -> Logical Operator/1
  Relational Operator/1 -> Logical Operator/2

== system BaseEngineController_LS/Foreground/Control/VirtualSensors/RawProcessed/VSPD_Selector ==
  VSPD_Dig : Inport
  VSPD_GPS : Inport  Port=2
  VSPD_GPSValid : Inport  Port=3
  Constant : Constant  Value=0
  Constant1 : Constant  Value=0
  Logical Operator : Logic  Inputs=3  AllPortsSameDT=off  OutDataTypeStr=boolean
  Logical Operator1 : Logic  Operator=NOT  AllPortsSameDT=off  OutDataTypeStr=boolean
  Logical Operator2 : Logic  Operator=NOT  AllPortsSameDT=off  OutDataTypeStr=boolean
  Logical Operator3 : Logic  AllPortsSameDT=off  OutDataTypeStr=boolean
  Switch : Switch  Criteria=u2 ~= 0
  Switch1 : Switch  Criteria=u2 ~= 0
  Switch2 : Switch  Criteria=u2 ~= 0
  motohawk_calibration : MotoHawk_lib/Calibration & Probing Blocks/motohawk_calibration  nam='VSPD_DigitalPresent'  val=1  storage=Calibration  show_more=on  name_source=Use Parameter  data_type=boolean  read_level=1  write_level=1  ovr_cals=on  view_as=Enumeration  enum_struct={'Disabled', 'Enabled'}  vector_style=Wide Row  use_help_units=off  help=''  units=''  use_header_enum=off  row_header_enum={}  col_header_enum={}  use_min_max=off  min_val=-inf  max_val=inf  use_precision=off  precision=''  gain=1  offset=0  exp=1  use_mototune_group=off  mototune_group=motohawk_vardec_path(gcb)
  motohawk_calibration1 : MotoHawk_lib/Calibration & Probing Blocks/motohawk_calibration  nam='VSPD_GPSPreferred'  val=1  storage=Calibration  show_more=on  name_source=Use Parameter  data_type=boolean  read_level=1  write_level=1  ovr_cals=on  view_as=Enumeration  enum_struct={'Disabled', 'Enabled'}  vector_style=Wide Row  use_help_units=off  help=''  units=''  use_header_enum=off  row_header_enum={}  col_header_enum={}  use_min_max=off  min_val=-inf  max_val=inf  use_precision=off  precision=''  gain=1  offset=0  exp=1  use_mototune_group=off  mototune_group=motohawk_vardec_path(gcb)
  motohawk_fault_status1 : MotoHawk_lib/Fault Management Blocks/motohawk_fault_status  source=Lookup By Name  nam='GPS_SpeedDir_Timeout'  status=Active
  motohawk_fault_status2 : MotoHawk_lib/Fault Management Blocks/motohawk_fault_status  source=Lookup By Name  nam='GPS_DateTime_Timeout'  status=Active
  motohawk_probe : MotoHawk_lib/Calibration & Probing Blocks/motohawk_probe  nam='VSPD_FinalFinal'  show_more=off  name_source=Use Parameter  read_level=1  view_as=Number  enum_struct={'Disabled', 'Enabled'}  vector_style=Wide Row  use_help_units=off  help=''  units=''  use_header_enum=off  row_header_enum={}  col_header_enum={}  use_precision=off  precision=''  gain=1  offset=0  exp=1  use_mototune_group=off  mototune_group=motohawk_vardec_path(gcb)
  VSPD_Final : Outport
  wires:
  motohawk_calibration/1 -> Switch/2
  VSPD_Dig/1 -> Switch/1
  Constant/1 -> Switch/3
  VSPD_GPSValid/1 -> Logical Operator/1
  motohawk_fault_status2/1 -> Logical Operator1/1
  motohawk_fault_status1/1 -> Logical Operator2/1
  Logical Operator1/1 -> Logical Operator/2
  Logical Operator2/1 -> Logical Operator/3
  Constant1/1 -> Switch1/3
  Logical Operator/1 -> Switch1/2, Logical Operator3/2
  VSPD_GPS/1 -> Switch1/1
  Logical Operator3/1 -> Switch2/2
  Switch1/1 -> Switch2/1
  motohawk_calibration1/1 -> Logical Operator3/1
  Switch/1 -> Switch2/3
  Switch2/1 -> VSPD_Final/1, motohawk_probe/1

== system BaseEngineController_LS/Foreground/Control/VirtualSensors/Virtual Indexes/ECT_KeyUp ==
  ECT_KeyUp : Inport
  motohawk_prelookup : MotoHawk_lib/Lookup Tables/motohawk_prelookup  nam='ECT_KeyUp09'  breakpoint_data=[-20 0 20 40 80 90 100 110 120]  show_more=on  data_type=Inherit from 'Table Data'  storage=Constant  read_level=1  write_level=1  ovr_cals=on  use_help=on  help='Index of ECT captured at key-up.'  units='degC'  use_min_max=off  min_val=-inf  max_val=inf  use_precision=on  precision=''  gain=1  offset=0  exp=1  use_links=on  input_name=''  use_mototune_group=on  mototune_group=motohawk_vardec_path(gcb)
  ECT_KeyUp09Idx : Outport
  wires:
  motohawk_prelookup/1 -> ECT_KeyUp09Idx/1
  ECT_KeyUp/1 -> motohawk_prelookup/1

== system BaseEngineController_LS/Foreground/Control/VirtualSensors/Virtual Indexes/IAT_KeyUp ==
  IAT_KeyUp : Inport
  motohawk_prelookup : MotoHawk_lib/Lookup Tables/motohawk_prelookup  nam='IAT_KeyUp09'  breakpoint_data=[-20 0 20 40 80 90 100 110 120]  show_more=on  data_type=Inherit from 'Table Data'  storage=Constant  read_level=1  write_level=1  ovr_cals=on  use_help=on  help='Index of IAT captured at key-up.'  units='degC'  use_min_max=off  min_val=-inf  max_val=inf  use_precision=on  precision=''  gain=1  offset=0  exp=1  use_links=on  input_name=''  use_mototune_group=on  mototune_group=motohawk_vardec_path(gcb)
  IAT_KeyUp09Idx : Outport
  wires:
  motohawk_prelookup/1 -> IAT_KeyUp09Idx/1
  IAT_KeyUp/1 -> motohawk_prelookup/1

== system BaseEngineController_LS/Foreground/Control/VirtualSensors/Virtual Indexes/MAFPortIndex ==
  MAFPort : Inport
  motohawk_prelookup : MotoHawk_lib/Lookup Tables/motohawk_prelookup  nam='MAFPort05'  breakpoint_data=[2 4 8 16 32]  show_more=on  data_type=Inherit from 'Table Data'  storage=Constant  read_level=1  write_level=1  ovr_cals=on  use_help=on  help='Index of MAF'  units='g/s'  use_min_max=on  min_val=0  max_val=1000000  use_precision=on  precision=''  gain=1  offset=0  exp=1  use_links=off  input_name=''  use_mototune_group=on  mototune_group=motohawk_vardec_path(gcb)
  MAFPort05Idx : Outport
  wires:
  MAFPort/1 -> motohawk_prelookup/1
  motohawk_prelookup/1 -> MAFPort05Idx/1

== system BaseEngineController_LS/Foreground/Inputs/Digital/Scramble /Button Delay 1 ==
  In1 : Inport
  Time : Inport  Port=2
  Logical Operator : Logic  AllPortsSameDT=off  OutDataTypeStr=boolean
  Relational Operator : RelationalOperator  OutDataTypeStr=boolean
  Time Since Enabled (With Input)4 : motohawk_control_primitives_lib/Time Since Enabled (With Input)1  SystemSampleTime=-1  nam='ScrambleDelay'  samp_time=-1  init=0  upperlim=3600*24
  Out1 : Outport
  wires:
  In1/1 -> Time Since Enabled (With Input)4/1, Logical Operator/1
  Time Since Enabled (With Input)4/1 -> Relational Operator/1
  Time/1 -> Relational Operator/2
  Relational Operator/1 -> Logical Operator/2
  Logical Operator/1 -> Out1/1

== system BaseEngineController_LS/Foreground/Inputs/EngineSpeed/Encoder Diagnostics/motohawk_model_probe_eval_f ==
  note: Simple Model Probe
  f : TriggerPort  TriggerType=function-call  ZeroCross=off
  Constant : Constant  Value=uint32(1)
  Sum : Sum  Inputs=|++
  Unit Delay : UnitDelay  SampleTime=-1
  motohawk_code_coverage : MotoHawk_lib/Extra Development Blocks/motohawk_code_coverage
  motohawk_probe : MotoHawk_lib/Calibration & Probing Blocks/motohawk_probe  nam=nam  show_more=on  name_source=Use Parameter  read_level=1  view_as=Number  enum_struct={'Disabled', 'Enabled'}  vector_style=Wide Row  use_help_units=off  help=''  units=''  use_header_enum=off  row_header_enum={}  col_header_enum={}  use_precision=off  precision=''  gain=1  offset=0  exp=1  use_mototune_group=on  mototune_group=group
  Count : Outport
  wires:
  Constant/1 -> Sum/1
  Unit Delay/1 -> Sum/2
  Sum/1 -> motohawk_probe/1, Count/1, Unit Delay/1

== system BaseEngineController_LS/Foreground/Inputs/LinearSensors/FuelOxygenationSensor/Filter Options ==
  In1 : Inport
  First Order Low Pass : motohawk_control_primitives_lib/First Order Low Pass (Tunable)  SystemSampleTime=-1  nam=[prefix 'FilterConst']  samp_time=samp_time  group=[group ' | ' nam ' Config']
  Moving Average Filter : Subsystem
  Multiport Switch : MultiPortSwitch  DataPortOrder=Zero-based contiguous  zeroidx=on
  Rate Limiter : Subsystem
  motohawk_calibration : MotoHawk_lib/Calibration & Probing Blocks/motohawk_calibration  nam='Filter_Type_Selection'  val=0  storage=Calibration  show_more=on  name_source=Use Parameter  data_type=uint8  read_level=1  write_level=1  ovr_cals=on  view_as=Enumeration  enum_struct={'Rate Limiter', 'Low Pass', 'Moving Average'}  vector_style=Wide Row  use_help_units=on  help='Filter Section For Fuel Oxygenation Sensor'  units=''  use_header_enum=off  row_header_enum={}  col_header_enum={}  use_min_max=off  min_val=-inf  max_val=inf  use_precision=on  precision=''  gain=1  offset=0  exp=1  use_mototune_group=on  mototune_group=motohawk_vardec_path(gcb)
  Out1 : Outport
  wires:
  In1/1 -> First Order Low Pass/1, Moving Average Filter/1(In1), Rate Limiter/1(In1)
  Moving Average Filter/1(Out1) -> Multiport Switch/4
  First Order Low Pass/1 -> Multiport Switch/3
  Rate Limiter/1(Out1) -> Multiport Switch/2
  motohawk_calibration/1 -> Multiport Switch/1
  Multiport Switch/1 -> Out1/1

== system BaseEngineController_LS/Foreground/Inputs/LinearSensors/FuelOxygenationSensor/If Action Subsystem ==
  In : Inport
  Action Port : ActionPort  ActionType=then
  Out : Outport
  wires:
  In/1 -> Out/1

== system BaseEngineController_LS/Foreground/Inputs/LinearSensors/FuelOxygenationSensor/If Action Subsystem1 ==
  In : Inport
  Action Port : ActionPort  ActionType=elseif
  Out : Outport
  wires:
  In/1 -> Out/1

== system BaseEngineController_LS/Foreground/Inputs/LinearSensors/FuelOxygenationSensor/If Action Subsystem2 ==
  In : Inport
  Action Port : ActionPort  ActionType=else
  Out : Outport
  wires:
  In/1 -> Out/1

== system BaseEngineController_LS/Foreground/Inputs/LinearSensors/MAP_Crank_Synchronous/MID_TDC ==
  f : TriggerPort  TriggerType=function-call
  Data Type Conversion : DataTypeConversion  SaturateOnIntegerOverflow=on  RndMeth=Zero
  motohawk_ain_read : MotoHawk_lib/Analog I//O Blocks/motohawk_ain_read  nam='MAPSensorPin'  typ=uint16
  ADC : Outport
  wires:
  motohawk_ain_read/1 -> Data Type Conversion/1
  Data Type Conversion/1 -> ADC/1

== system BaseEngineController_LS/Foreground/Inputs/LinearSensors/MAP_Crank_Synchronous/Once at Startup ==
  note: Sample Crank-Synchronous MAP Once at Startup
  f : TriggerPort  TriggerType=function-call
  Data Type Conversion : DataTypeConversion  SaturateOnIntegerOverflow=on  RndMeth=Zero
  motohawk_ain : MotoHawk_lib/Analog I//O Blocks/motohawk_ain  res_name=[]  text_resource=AN1M  code_resource=RES_ECUP  val_resource=-1  target=ECU555-80  resource_enum_str=(None)=-1,ECUP=53,DRVP=54,XDRP=55,AN1M=56,AN2M=57,AN3M=58,AN4M=59,AN5M=60,AN6M=61,AN7M=62,AN8M=63,AN9M=64,AN10M=65,AN11M=66,AN12M=67,AN13M=68,AN14M=69,AN15M=70,AN16M=71,AN17M=72,AN18M=73,AN19M=74,O2A=90,O2B=91,XDRP_B=92  altref=5V Reference  typ=uint16  num_adc_bits=10  use_stat=off  use_vardec=on  nam='MAPSensorPin'  read_level=1  write_level=1  group='System | I/O Pins | Inputs Config'
  ADC : Outport
  wires:
  Data Type Conversion/1 -> ADC/1
  motohawk_ain/1 -> Data Type Conversion/1

== system BaseEngineController_LS/Foreground/Inputs/PotentiometerSensors/APP1/If Action Subsystem ==
  In : Inport
  Action Port : ActionPort  ActionType=then
  Out : Outport
  wires:
  In/1 -> Out/1

== system BaseEngineController_LS/Foreground/Inputs/PotentiometerSensors/APP1/If Action Subsystem1 ==
  In : Inport
  Action Port : ActionPort  ActionType=elseif
  Out : Outport
  wires:
  In/1 -> Out/1

== system BaseEngineController_LS/Foreground/Inputs/PotentiometerSensors/APP1/If Action Subsystem2 ==
  In : Inport
  Action Port : ActionPort  ActionType=else
  Out : Outport
  wires:
  In/1 -> Out/1

== system BaseEngineController_LS/Foreground/Inputs/PotentiometerSensors/APP1ForcedAdapt/Function-Call Subsystem ==
  function : TriggerPort  TriggerType=function-call
  First Time : motohawk_control_primitives_lib/First Time  SystemSampleTime=-1
  Logical Operator : Logic  Operator=OR  AllPortsSameDT=off  OutDataTypeStr=boolean
  motohawk_calibration : MotoHawk_lib/Calibration & Probing Blocks/motohawk_calibration  nam='APP1_AlwaysAdapt'  val=0  storage=Calibration  show_more=on  name_source=Use Parameter  data_type=boolean  read_level=1  write_level=1  ovr_cals=on  view_as=Enumeration  enum_struct={'Disabled', 'Enabled'}  vector_style=Wide Row  use_help_units=off  help=''  units=''  use_header_enum=off  row_header_enum={}  col_header_enum={}  use_min_max=off  min_val=-inf  max_val=inf  use_precision=off  precision=''  gain=1  offset=0  exp=1  use_mototune_group=off  mototune_group=motohawk_vardec_path(gcb)
  Out1 : Outport  InitialOutput=false
  wires:
  First Time/1 -> Logical Operator/1
  motohawk_calibration/1 -> Logical Operator/2
  Logical Operator/1 -> Out1/1

== system BaseEngineController_LS/Foreground/Inputs/PotentiometerSensors/APP2/If Action Subsystem ==
  In : Inport
  Action Port : ActionPort  ActionType=then
  Out : Outport
  wires:
  In/1 -> Out/1

== system BaseEngineController_LS/Foreground/Inputs/PotentiometerSensors/APP2/If Action Subsystem1 ==
  In : Inport
  Action Port : ActionPort  ActionType=elseif
  Out : Outport
  wires:
  In/1 -> Out/1

== system BaseEngineController_LS/Foreground/Inputs/PotentiometerSensors/APP2/If Action Subsystem2 ==
  In : Inport
  Action Port : ActionPort  ActionType=else
  Out : Outport
  wires:
  In/1 -> Out/1
